simulink model "model"  (R2021b)
settings: Solver=FixedStepAuto  StartTime=0.0  StopTime=100  FixedStep=0.05  RelTol=1e-3
undefined symbols (not defined in the file): A, parameters, waypoints, waypoints_K
libraries: mssSimulink x9
settings Model: Creator=simengangstad  LastModifiedBy=simengangstad

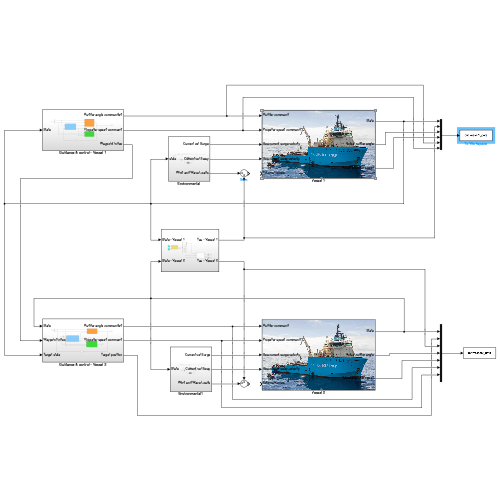
[thumbnail: Simulink's stored preview of the top-level diagram]
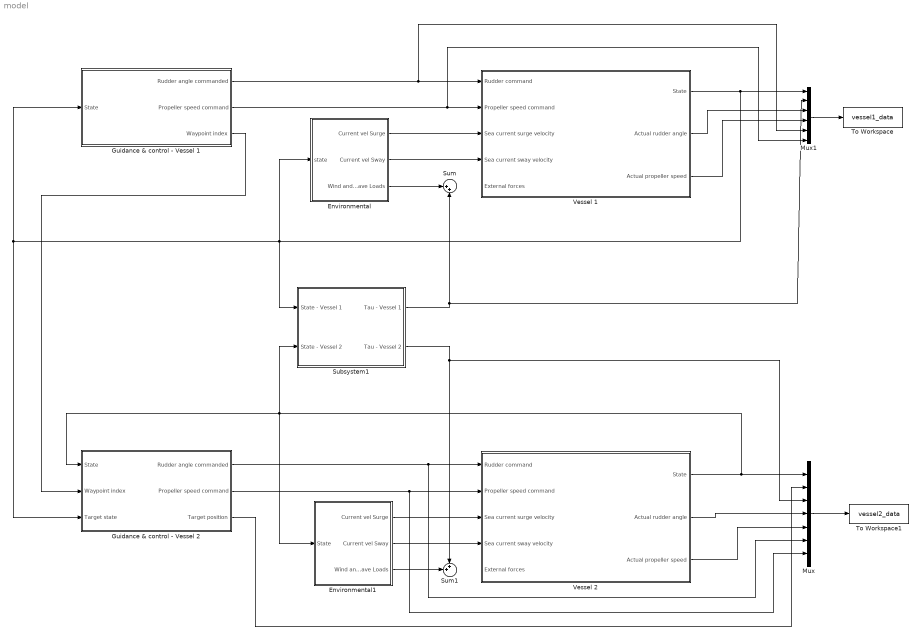
== system model ==
  Environmental : Subsystem
  Environmental1 : Subsystem
  Guidance & control - Vessel 1 : Subsystem
  Guidance & control - Vessel 2 : Subsystem
  Mux : Mux  Inputs=7
  Mux1 : Mux  Inputs=6
  Subsystem1 : Subsystem
  Sum : Sum  Inputs=|++
  Sum1 : Sum  Inputs=++|
  To Workspace : ToWorkspace  VariableName=vessel1_data  SaveFormat=Timeseries  SampleTime=-1
  To Workspace1 : ToWorkspace  VariableName=vessel2_data  SaveFormat=Timeseries  SampleTime=-1
  Vessel 1 : Subsystem
      mask Display: image('$imagefile'); % Use "Edit Image" on toolstrip to change.
  Vessel 2 : Subsystem
      mask Display: image('$imagefile'); % Use "Edit Image" on toolstrip to change.
  wires:
  Vessel 1/1(State) -> Environmental/1(state), Guidance & control - Vessel 1/1(State), Guidance & control - Vessel 2/3(Target state), Subsystem1/1(State - Vessel 1), Mux1/1
  Vessel 1/2(Actual rudder angle) -> Mux1/3
  Vessel 1/3(Actual propeller speed) -> Mux1/4
  Environmental/2(Current vel Sway) -> Vessel 1/4(Sea current sway velocity)
  Environmental/1(Current vel Surge) -> Vessel 1/3(Sea current surge velocity)
  Environmental1/1(Current vel Surge) -> Vessel 2/3(Sea current surge velocity)
  Environmental1/2(Current vel Sway) -> Vessel 2/4(Sea current sway velocity)
  Vessel 2/2(Actual rudder angle) -> Mux/4
  Vessel 2/3(Actual propeller speed) -> Mux/5
  Mux/1 -> To Workspace1/1
  Guidance & control - Vessel 1/1(Rudder angle commanded) -> Mux1/5, Vessel 1/1(Rudder command)
  Guidance & control - Vessel 1/2(Propeller speed command) -> Mux1/6, Vessel 1/2(Propeller speed command)
  Guidance & control - Vessel 1/3(Waypoint index) -> Guidance & control - Vessel 2/2(Waypoint index)
  Guidance & control - Vessel 2/1(Rudder angle commanded) -> Mux/6, Vessel 2/1(Rudder command)
  Guidance & control - Vessel 2/2(Propeller speed command) -> Mux/7, Vessel 2/2(Propeller speed command)
  Guidance & control - Vessel 2/3(Target position) -> Mux/2
  Vessel 2/1(State) -> Subsystem1/2(State - Vessel 2), Guidance & control - Vessel 2/1(State), Environmental1/1(State), Mux/1
  Subsystem1/1(Tau - Vessel 1) -> Sum/2, Mux1/2
  Environmental/3(Wind and Wave Loads) -> Sum/1
  Environmental1/3(Wind and Wave Loads) -> Sum1/2
  Subsystem1/2(Tau - Vessel 2) -> Sum1/1, Mux/3
  Mux1/1 -> To Workspace/1

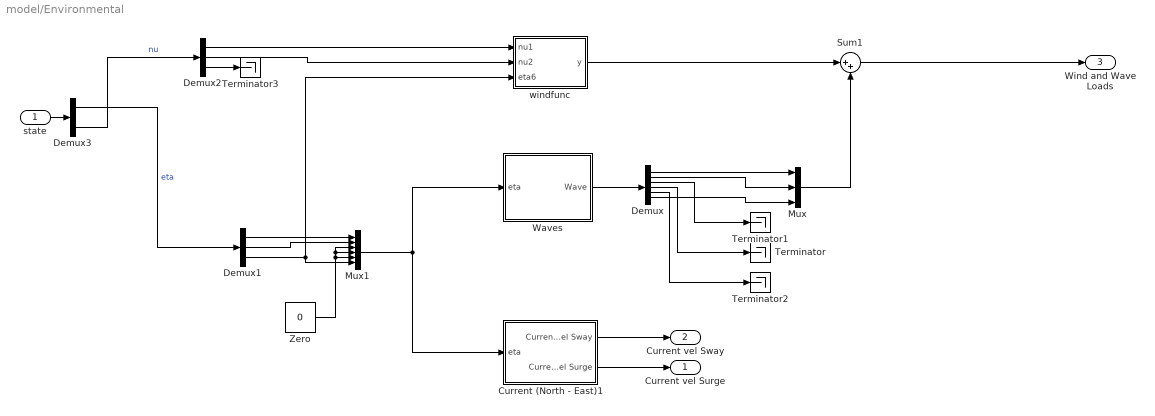
== system model/Environmental ==
  state : Inport
  Current (North - East)1 : Subsystem
  Demux : Demux  Outputs=6
  Demux1 : Demux  Outputs=3
  Demux2 : Demux  Outputs=3
  Demux3 : Demux  Outputs=2
  Mux : Mux  Inputs=3
  Mux1 : Mux  Inputs=6
  Sum1 : Sum  Inputs=|++
  Terminator{,1..3} (4 alike) : Terminator
  Waves : Subsystem
  Zero : Constant  Value=0  OutDataTypeStr=Inherit: Inherit via back propagation
  windfunc : MATLAB Function  TreatAsAtomicUnit=on
  Current vel Surge : Outport
  Current vel Sway : Outport  Port=2
  Wind and Wave Loads : Outport  Port=3
  wires:
  Demux/1 -> Mux/1
  Demux/2 -> Mux/2
  Demux/6 -> Mux/3
  Demux/3 -> Terminator1/1
  Demux/4 -> Terminator/1
  Demux/5 -> Terminator2/1
  Demux3/1 -> Demux1/1  "eta"
  Demux1/1 -> Mux1/1
  Demux1/2 -> Mux1/2
  Demux1/3 -> Mux1/6, windfunc/3(eta6)
  Zero/1 -> Mux1/5, Mux1/4, Mux1/3
  Mux1/1 -> Current (North - East)1/1(eta), Waves/1(eta)
  Waves/1(Wave) -> Demux/1
  windfunc/1(y) -> Sum1/1
  Demux3/2 -> Demux2/1  "nu"
  Demux2/1 -> windfunc/1(nu1)
  Demux2/2 -> windfunc/2(nu2)
  Demux2/3 -> Terminator3/1
  Mux/1 -> Sum1/2
  Sum1/1 -> Wind and Wave Loads/1
  Current (North - East)1/1(Currentvel Sway) -> Current vel Sway/1
  Current (North - East)1/2(Currentvel Surge) -> Current vel Surge/1
  state/1 -> Demux3/1

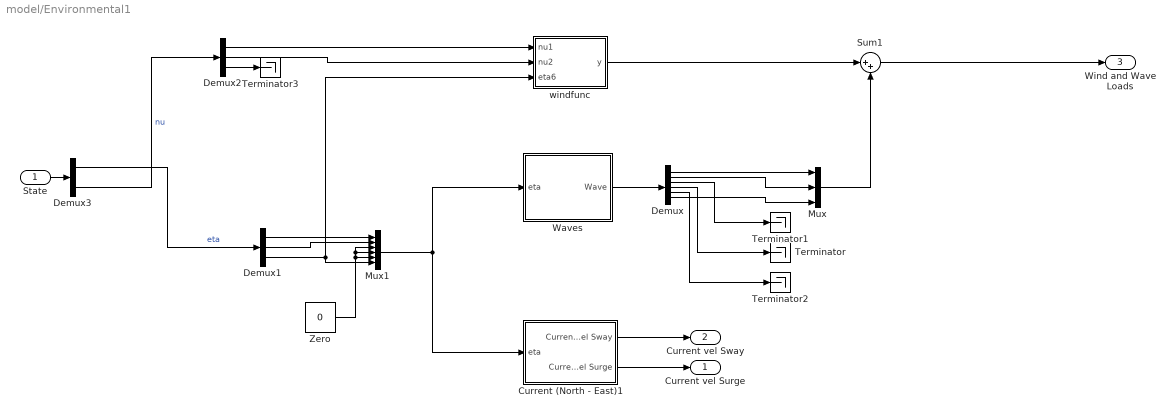
== system model/Environmental1 ==
  State : Inport
  Current (North - East)1 : Subsystem
  Demux : Demux  Outputs=6
  Demux1 : Demux  Outputs=3
  Demux2 : Demux  Outputs=3
  Demux3 : Demux  Outputs=2
  Mux : Mux  Inputs=3
  Mux1 : Mux  Inputs=6
  Sum1 : Sum  Inputs=|++
  Terminator{,1..3} (4 alike) : Terminator
  Waves : Subsystem
  Zero : Constant  Value=0  OutDataTypeStr=Inherit: Inherit via back propagation
  windfunc : MATLAB Function  TreatAsAtomicUnit=on
  Current vel Surge : Outport
  Current vel Sway : Outport  Port=2
  Wind and Wave Loads : Outport  Port=3
  wires:
  Demux/1 -> Mux/1
  Demux/2 -> Mux/2
  Demux/6 -> Mux/3
  Demux/3 -> Terminator1/1
  Demux/4 -> Terminator/1
  Demux/5 -> Terminator2/1
  Demux3/1 -> Demux1/1  "eta"
  Demux1/1 -> Mux1/1
  Demux1/2 -> Mux1/2
  Demux1/3 -> Mux1/6, windfunc/3(eta6)
  Zero/1 -> Mux1/5, Mux1/4, Mux1/3
  Mux1/1 -> Current (North - East)1/1(eta), Waves/1(eta)
  Waves/1(Wave) -> Demux/1
  windfunc/1(y) -> Sum1/1
  Demux3/2 -> Demux2/1  "nu"
  Demux2/1 -> windfunc/1(nu1)
  Demux2/2 -> windfunc/2(nu2)
  Demux2/3 -> Terminator3/1
  Mux/1 -> Sum1/2
  Sum1/1 -> Wind and Wave Loads/1
  Current (North - East)1/1(Currentvel Sway) -> Current vel Sway/1
  Current (North - East)1/2(Currentvel Surge) -> Current vel Surge/1
  State/1 -> Demux3/1

== system model/Guidance & control - Vessel 1 ==
  State : Inport
  Constant : Constant  Value=1.5
  Demux1 : Demux  Outputs=2
  Guidance : Subsystem
  Heading controller : Subsystem
  Memory : Memory
  Speed controller : Subsystem
  Rudder angle commanded : Outport
  Propeller speed command : Outport  Port=2
  Waypoint index : Outport  Port=3
  wires:
  Demux1/2 -> Speed controller/2(nu), Heading controller/2(nu)
  Guidance/2(Waypoint index) -> Waypoint index/1, Speed controller/3(Waypoint index)
  Speed controller/1(Propeller speed command) -> Propeller speed command/1
  Constant/1 -> Speed controller/1(Speed reference)
  Guidance/1(psi_ref) -> Heading controller/3(psi_ref)
  Demux1/1 -> Guidance/1(eta), Heading controller/1(eta)
  Memory/1 -> Guidance/2(Rudder angle commanded)
  Heading controller/1(Rudder angle commanded) -> Rudder angle commanded/1, Memory/1
  State/1 -> Demux1/1

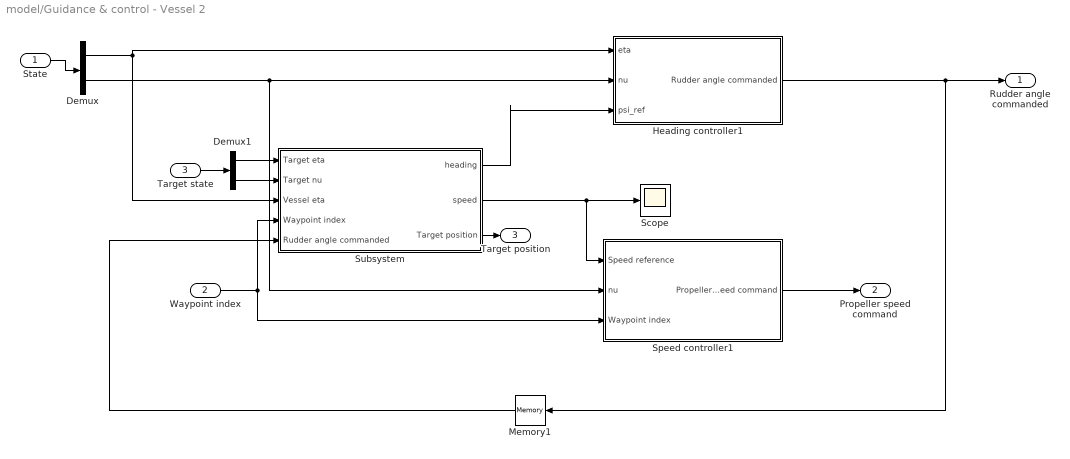
== system model/Guidance & control - Vessel 2 ==
  State : Inport
  Waypoint index : Inport  Port=2
  Target state : Inport  Port=3
  Demux : Demux  Outputs=2
  Demux1 : Demux  Outputs=2
  Heading controller1 : Subsystem
  Memory1 : Memory
  Scope : Scope
  Speed controller1 : Subsystem
  Subsystem : Subsystem
  Rudder angle commanded : Outport
  Propeller speed command : Outport  Port=2
  Target position : Outport  Port=3
  wires:
  Demux1/2 -> Subsystem/2(Target nu)
  Demux1/1 -> Subsystem/1(Target eta)
  Speed controller1/1(Propeller speed command) -> Propeller speed command/1
  Subsystem/3(Target position) -> Target position/1
  Waypoint index/1 -> Subsystem/4(Waypoint index), Speed controller1/3(Waypoint index)
  Memory1/1 -> Subsystem/5(Rudder angle commanded)
  Subsystem/2(speed) -> Scope/1, Speed controller1/1(Speed reference)
  Demux/1 -> Heading controller1/1(eta), Subsystem/3(Vessel eta)
  Subsystem/1(heading) -> Heading controller1/3(psi_ref)
  Demux/2 -> Heading controller1/2(nu), Speed controller1/2(nu)
  Heading controller1/1(Rudder angle commanded) -> Memory1/1, Rudder angle commanded/1
  State/1 -> Demux/1
  Target state/1 -> Demux1/1

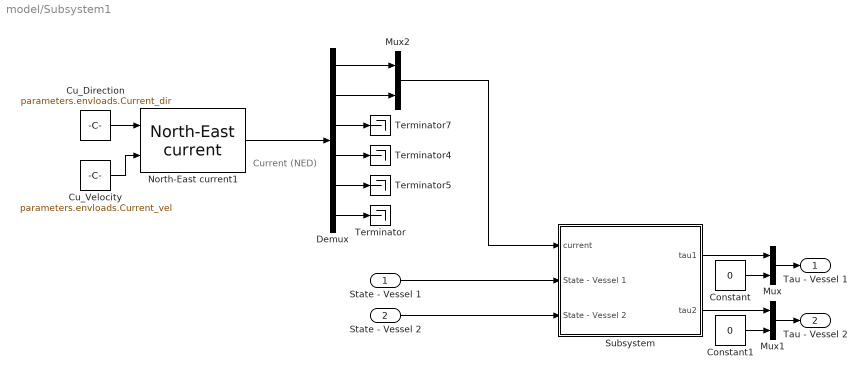
== system model/Subsystem1 ==
  note: Current (NED)
  State - Vessel 1 : Inport
  State - Vessel 2 : Inport  Port=2
  Constant : Constant  Value=0
  Constant1 : Constant  Value=0
  Cu_Direction : Constant  Value=parameters.envloads.Current_dir
  Cu_Velocity : Constant  Value=parameters.envloads.Current_vel
  Demux : Demux  Outputs=6
  Mux : Mux  Inputs=2
  Mux1 : Mux  Inputs=2
  Mux2 : Mux  Inputs=2
  North-East current1 : mssSimulink/Environment/Current/North-East current  SystemSampleTime=-1  VariantActivationTime=update diagram  Latency=0  AutoFrameSizeCalculation=off
  Subsystem : Subsystem
  Terminator{,4..5,7} (4 alike) : Terminator
  Tau - Vessel 1 : Outport
  Tau - Vessel 2 : Outport  Port=2
  wires:
  Demux/6 -> Terminator/1
  Demux/4 -> Terminator4/1
  Demux/1 -> Mux2/1
  North-East current1/1 -> Demux/1
  State - Vessel 1/1 -> Subsystem/2(State - Vessel 1)
  Cu_Direction/1 -> North-East current1/1
  State - Vessel 2/1 -> Subsystem/3(State - Vessel 2)
  Demux/3 -> Terminator7/1
  Mux2/1 -> Subsystem/1(current)
  Cu_Velocity/1 -> North-East current1/2
  Demux/2 -> Mux2/2
  Demux/5 -> Terminator5/1
  Mux/1 -> Tau - Vessel 1/1
  Subsystem/1(tau1) -> Mux/1
  Constant/1 -> Mux/2
  Mux1/1 -> Tau - Vessel 2/1
  Subsystem/2(tau2) -> Mux1/1
  Constant1/1 -> Mux1/2

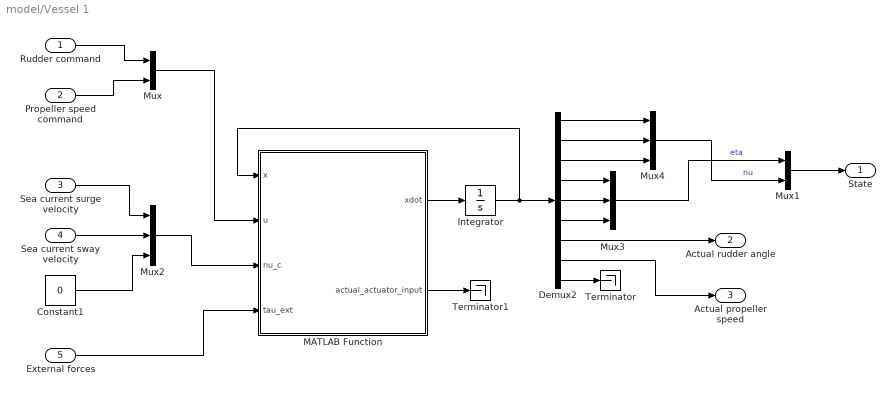
== system model/Vessel 1 ==
  Rudder command : Inport
  Propeller speed command : Inport  Port=2
  Sea current surge velocity : Inport  Port=3
  Sea current sway velocity : Inport  Port=4
  External forces : Inport  Port=5
  Constant1 : Constant  Value=0
  Demux2 : Demux  Outputs=9
  Integrator : Integrator  InitialCondition=[0, 0, 0, 0, 0, pi/2, 0, 0, 0]
  MATLAB Function : MATLAB Function  TreatAsAtomicUnit=on
  Mux : Mux  Inputs=2
  Mux1 : Mux  Inputs=2
  Mux2 : Mux  Inputs=3
  Mux3 : Mux  Inputs=3
  Mux4 : Mux  Inputs=3
  Terminator : Terminator
  Terminator1 : Terminator
  State : Outport
  Actual rudder angle : Outport  Port=2
  Actual propeller speed : Outport  Port=3
  wires:
  Demux2/3 -> Mux4/3
  Demux2/7 -> Actual rudder angle/1
  Mux/1 -> MATLAB Function/2(u)
  External forces/1 -> MATLAB Function/4(tau_ext)
  Mux2/1 -> MATLAB Function/3(nu_c)
  Mux4/1 -> Mux1/2  "nu"
  MATLAB Function/1(xdot) -> Integrator/1
  Propeller speed command/1 -> Mux/2
  Demux2/4 -> Mux3/1
  Demux2/5 -> Mux3/2
  Sea current surge velocity/1 -> Mux2/1
  Constant1/1 -> Mux2/3
  Sea current sway velocity/1 -> Mux2/2
  Mux3/1 -> Mux1/1  "eta"
  Demux2/2 -> Mux4/2
  Demux2/8 -> Actual propeller speed/1
  Demux2/1 -> Mux4/1
  Integrator/1 -> MATLAB Function/1(x), Demux2/1
  Rudder command/1 -> Mux/1
  Demux2/6 -> Mux3/3
  Demux2/9 -> Terminator/1
  MATLAB Function/2(actual_actuator_input) -> Terminator1/1
  Mux1/1 -> State/1

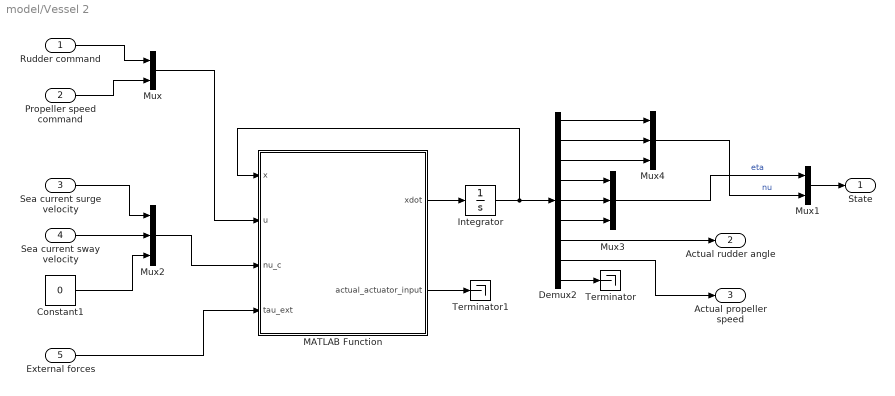
== system model/Vessel 2 ==
  Rudder command : Inport
  Propeller speed command : Inport  Port=2
  Sea current surge velocity : Inport  Port=3
  Sea current sway velocity : Inport  Port=4
  External forces : Inport  Port=5
  Constant1 : Constant  Value=0
  Demux2 : Demux  Outputs=9
  Integrator : Integrator  InitialCondition=[0, 0, 0, 500, 0, pi/2, 0, 0, 0]
  MATLAB Function : MATLAB Function  TreatAsAtomicUnit=on
  Mux : Mux  Inputs=2
  Mux1 : Mux  Inputs=2
  Mux2 : Mux  Inputs=3
  Mux3 : Mux  Inputs=3
  Mux4 : Mux  Inputs=3
  Terminator : Terminator
  Terminator1 : Terminator
  State : Outport
  Actual rudder angle : Outport  Port=2
  Actual propeller speed : Outport  Port=3
  wires:
  Demux2/3 -> Mux4/3
  Demux2/7 -> Actual rudder angle/1
  Mux/1 -> MATLAB Function/2(u)
  External forces/1 -> MATLAB Function/4(tau_ext)
  Mux2/1 -> MATLAB Function/3(nu_c)
  Mux4/1 -> Mux1/2  "nu"
  MATLAB Function/1(xdot) -> Integrator/1
  Propeller speed command/1 -> Mux/2
  Demux2/4 -> Mux3/1
  Demux2/5 -> Mux3/2
  Sea current surge velocity/1 -> Mux2/1
  Constant1/1 -> Mux2/3
  Sea current sway velocity/1 -> Mux2/2
  Mux3/1 -> Mux1/1  "eta"
  Demux2/2 -> Mux4/2
  Demux2/8 -> Actual propeller speed/1
  Demux2/1 -> Mux4/1
  Integrator/1 -> MATLAB Function/1(x), Demux2/1
  Rudder command/1 -> Mux/1
  Demux2/6 -> Mux3/3
  Demux2/9 -> Terminator/1
  MATLAB Function/2(actual_actuator_input) -> Terminator1/1
  Mux1/1 -> State/1

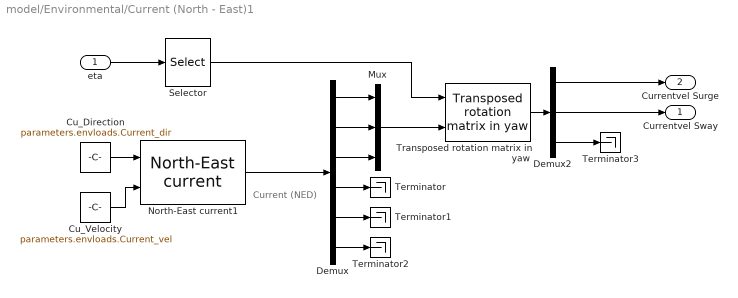
== system model/Environmental/Current (North - East)1 ==
  note: Current (NED)
  eta : Inport
  Cu_Direction : Constant  Value=parameters.envloads.Current_dir
  Cu_Velocity : Constant  Value=parameters.envloads.Current_vel
  Demux : Demux  Outputs=6
  Demux2 : Demux  Outputs=3
  Mux : Mux  Inputs=3
  North-East current1 : mssSimulink/Environment/Current/North-East current  SystemSampleTime=-1  VariantActivationTime=update diagram  Latency=0  AutoFrameSizeCalculation=off
  Selector : Selector  InputPortWidth=6  IndexOptions=Index vector (dialog)  Indices=[6]  OutputSizes=1
  Terminator{,1..3} (4 alike) : Terminator
  Transposed rotation matrix in yaw : mssSimulink/Modelling/Kinematics/Transposed rotation  matrix in yaw
  Currentvel Sway : Outport  VectorParamsAs1DForOutWhenUnconnected=off
  Currentvel Surge : Outport  Port=2
  wires:
  Demux/6 -> Terminator2/1
  North-East current1/1 -> Demux/1
  Demux/4 -> Terminator/1
  Demux/5 -> Terminator1/1
  Selector/1 -> Transposed rotation matrix in yaw/1
  Demux/3 -> Mux/3
  Mux/1 -> Transposed rotation matrix in yaw/2
  Demux/1 -> Mux/1
  Cu_Velocity/1 -> North-East current1/2
  Demux/2 -> Mux/2
  Demux2/2 -> Currentvel Sway/1
  Transposed rotation matrix in yaw/1 -> Demux2/1
  eta/1 -> Selector/1
  Cu_Direction/1 -> North-East current1/1
  Demux2/1 -> Currentvel Surge/1
  Demux2/3 -> Terminator3/1

== system model/Environmental/Waves ==
  eta : Inport
  Terminator : Terminator
  Wave generator : mssSimulink/Environment/Waves/Waves  spectrum_type=ITTC  disp_flag=on  plot_spectrum=off  plot_realization=off  hs=0.8  omega_peak=0  psi_mean=0  gamma=-1  spread=2  depth=inf  nfreq=20  ndir=10  energylim=0.005  freq_cutoff=3  dir_cutoff=0  rand_seed=123  rand_freq=on  rand_dir=on  Zeta_a=0  Omega=0  Phase=0  Wavenum=0  Psi=0
  WaveLoad : Subsystem  mask{waveforces=on}
      mask prompts: waveforces "Waveforces enabled"
  Wave : Outport  VectorParamsAs1DForOutWhenUnconnected=off
  wires:
  Wave generator/1 -> WaveLoad/2(waves)
  Wave generator/2 -> Terminator/1
  eta/1 -> WaveLoad/1(eta)
  WaveLoad/1(Wave) -> Wave/1

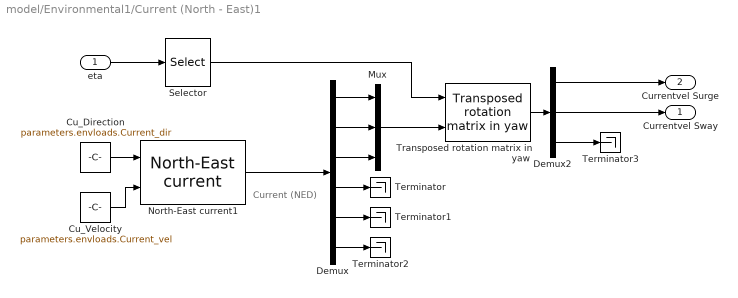
== system model/Environmental1/Current (North - East)1 ==
  note: Current (NED)
  eta : Inport
  Cu_Direction : Constant  Value=parameters.envloads.Current_dir
  Cu_Velocity : Constant  Value=parameters.envloads.Current_vel
  Demux : Demux  Outputs=6
  Demux2 : Demux  Outputs=3
  Mux : Mux  Inputs=3
  North-East current1 : mssSimulink/Environment/Current/North-East current  SystemSampleTime=-1  VariantActivationTime=update diagram  Latency=0  AutoFrameSizeCalculation=off
  Selector : Selector  InputPortWidth=6  IndexOptions=Index vector (dialog)  Indices=[6]  OutputSizes=1
  Terminator{,1..3} (4 alike) : Terminator
  Transposed rotation matrix in yaw : mssSimulink/Modelling/Kinematics/Transposed rotation  matrix in yaw
  Currentvel Sway : Outport  VectorParamsAs1DForOutWhenUnconnected=off
  Currentvel Surge : Outport  Port=2
  wires:
  Demux/6 -> Terminator2/1
  North-East current1/1 -> Demux/1
  Demux/4 -> Terminator/1
  Demux/5 -> Terminator1/1
  Selector/1 -> Transposed rotation matrix in yaw/1
  Demux/3 -> Mux/3
  Mux/1 -> Transposed rotation matrix in yaw/2
  Demux/1 -> Mux/1
  Cu_Velocity/1 -> North-East current1/2
  Demux/2 -> Mux/2
  Demux2/2 -> Currentvel Sway/1
  Transposed rotation matrix in yaw/1 -> Demux2/1
  eta/1 -> Selector/1
  Cu_Direction/1 -> North-East current1/1
  Demux2/1 -> Currentvel Surge/1
  Demux2/3 -> Terminator3/1

== system model/Environmental1/Waves ==
  eta : Inport
  Terminator : Terminator
  Wave generator : mssSimulink/Environment/Waves/Waves  spectrum_type=ITTC  disp_flag=on  plot_spectrum=off  plot_realization=off  hs=0.8  omega_peak=0  psi_mean=0  gamma=-1  spread=2  depth=inf  nfreq=20  ndir=10  energylim=0.005  freq_cutoff=3  dir_cutoff=0  rand_seed=123  rand_freq=on  rand_dir=on  Zeta_a=0  Omega=0  Phase=0  Wavenum=0  Psi=0
  WaveLoad : Subsystem  mask{waveforces=on}
      mask prompts: waveforces "Waveforces enabled"
  Wave : Outport  VectorParamsAs1DForOutWhenUnconnected=off
  wires:
  Wave generator/1 -> WaveLoad/2(waves)
  Wave generator/2 -> Terminator/1
  eta/1 -> WaveLoad/1(eta)
  WaveLoad/1(Wave) -> Wave/1

== system model/Guidance & control - Vessel 1/Guidance ==
  eta : Inport
  Rudder angle commanded : Inport  Port=2
  Demux2 : Demux  Outputs=3
  MATLAB Function : MATLAB Function  TreatAsAtomicUnit=on
  Terminator : Terminator
  psi_ref : Outport
  Waypoint index : Outport  Port=2
  wires:
  MATLAB Function/1(psi_ref) -> psi_ref/1
  eta/1 -> Demux2/1
  Rudder angle commanded/1 -> MATLAB Function/3(rudder_angle_commanded)
  Demux2/1 -> MATLAB Function/1(x)
  Demux2/2 -> MATLAB Function/2(y)
  Demux2/3 -> Terminator/1
  MATLAB Function/2(waypoint_idx) -> Waypoint index/1

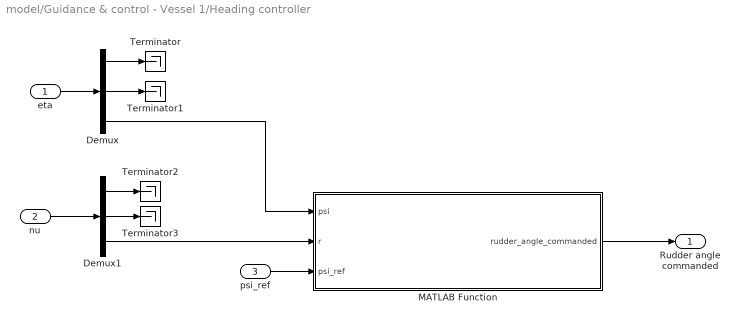
== system model/Guidance & control - Vessel 1/Heading controller ==
  eta : Inport
  nu : Inport  Port=2
  psi_ref : Inport  Port=3
  Demux : Demux  Outputs=3
  Demux1 : Demux  Outputs=3
  MATLAB Function : MATLAB Function  TreatAsAtomicUnit=on
  Terminator{,1..3} (4 alike) : Terminator
  Rudder angle commanded : Outport
  wires:
  MATLAB Function/1(rudder_angle_commanded) -> Rudder angle commanded/1
  Demux1/3 -> MATLAB Function/2(r)
  Demux/2 -> Terminator1/1
  psi_ref/1 -> MATLAB Function/3(psi_ref)
  Demux1/1 -> Terminator2/1
  Demux1/2 -> Terminator3/1
  Demux/3 -> MATLAB Function/1(psi)
  nu/1 -> Demux1/1
  eta/1 -> Demux/1
  Demux/1 -> Terminator/1

== system model/Guidance & control - Vessel 1/Speed controller ==
  Speed reference : Inport
  nu : Inport  Port=2
  Waypoint index : Inport  Port=3
  Demux2 : Demux  Outputs=3
  MATLAB Function : MATLAB Function  TreatAsAtomicUnit=on
  Terminator : Terminator
  Terminator1 : Terminator
  Propeller speed command : Outport
  wires:
  Demux2/1 -> MATLAB Function/1(u)
  Speed reference/1 -> MATLAB Function/2(U_ref)
  nu/1 -> Demux2/1
  MATLAB Function/1(n_c) -> Propeller speed command/1
  Demux2/2 -> Terminator/1
  Demux2/3 -> Terminator1/1
  Waypoint index/1 -> MATLAB Function/3(waypoint_index)

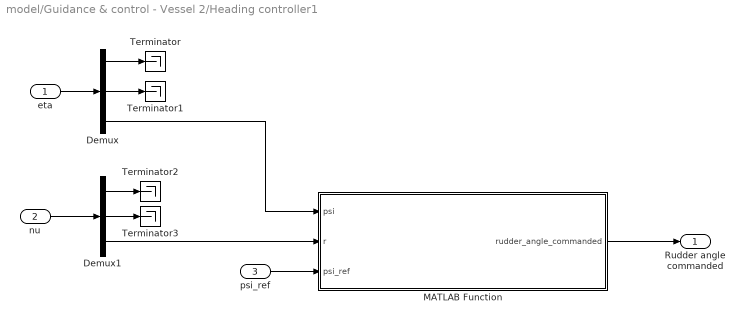
== system model/Guidance & control - Vessel 2/Heading controller1 ==
  eta : Inport
  nu : Inport  Port=2
  psi_ref : Inport  Port=3
  Demux : Demux  Outputs=3
  Demux1 : Demux  Outputs=3
  MATLAB Function : MATLAB Function  TreatAsAtomicUnit=on
  Terminator{,1..3} (4 alike) : Terminator
  Rudder angle commanded : Outport
  wires:
  MATLAB Function/1(rudder_angle_commanded) -> Rudder angle commanded/1
  psi_ref/1 -> MATLAB Function/3(psi_ref)
  Demux1/3 -> MATLAB Function/2(r)
  Demux/3 -> MATLAB Function/1(psi)
  eta/1 -> Demux/1
  nu/1 -> Demux1/1
  Demux/1 -> Terminator/1
  Demux/2 -> Terminator1/1
  Demux1/1 -> Terminator2/1
  Demux1/2 -> Terminator3/1

== system model/Guidance & control - Vessel 2/Speed controller1 ==
  Speed reference : Inport
  nu : Inport  Port=2
  Waypoint index : Inport  Port=3
  Demux2 : Demux  Outputs=3
  MATLAB Function : MATLAB Function  TreatAsAtomicUnit=on
  Terminator : Terminator
  Terminator1 : Terminator
  Propeller speed command : Outport
  wires:
  Demux2/1 -> MATLAB Function/1(u)
  Speed reference/1 -> MATLAB Function/2(U_ref)
  nu/1 -> Demux2/1
  MATLAB Function/1(n_c) -> Propeller speed command/1
  Demux2/2 -> Terminator/1
  Demux2/3 -> Terminator1/1
  Waypoint index/1 -> MATLAB Function/3(waypoint_index)

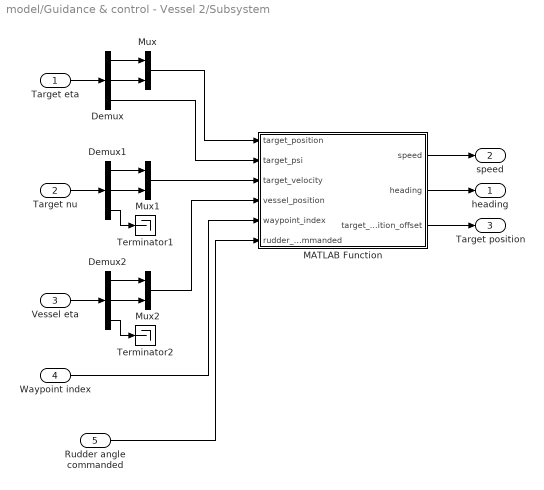
== system model/Guidance & control - Vessel 2/Subsystem ==
  Target eta : Inport
  Target nu : Inport  Port=2
  Vessel eta : Inport  Port=3
  Waypoint index : Inport  Port=4
  Rudder angle commanded : Inport  Port=5
  Demux : Demux  Outputs=3
  Demux1 : Demux  Outputs=3
  Demux2 : Demux  Outputs=3
  MATLAB Function : MATLAB Function  TreatAsAtomicUnit=on
  Mux : Mux  Inputs=2
  Mux1 : Mux  Inputs=2
  Mux2 : Mux  Inputs=2
  Terminator1 : Terminator
  Terminator2 : Terminator
  heading : Outport
  speed : Outport  Port=2
  Target position : Outport  Port=3
  wires:
  MATLAB Function/2(heading) -> heading/1
  MATLAB Function/1(speed) -> speed/1
  Demux/1 -> Mux/1
  Demux/2 -> Mux/2
  Demux/3 -> MATLAB Function/2(target_psi)
  Target eta/1 -> Demux/1
  Mux/1 -> MATLAB Function/1(target_position)
  Mux1/1 -> MATLAB Function/3(target_velocity)
  Demux1/1 -> Mux1/1
  Target nu/1 -> Demux1/1
  Demux1/3 -> Terminator1/1
  Demux1/2 -> Mux1/2
  Vessel eta/1 -> Demux2/1
  Demux2/2 -> Mux2/2
  Demux2/3 -> Terminator2/1
  Demux2/1 -> Mux2/1
  Mux2/1 -> MATLAB Function/4(vessel_position)
  Waypoint index/1 -> MATLAB Function/5(waypoint_index)
  MATLAB Function/3(target_position_offset) -> Target position/1
  Rudder angle commanded/1 -> MATLAB Function/6(rudder_angle_commanded)

== system model/Subsystem1/Subsystem ==
  current : Inport
  State - Vessel 1 : Inport  Port=2
  State - Vessel 2 : Inport  Port=3
  Attack velocity (B frame to net frame) : MATLAB Function  TreatAsAtomicUnit=on
  Demux : Demux  Outputs=2
  Demux1 : Demux  Outputs=2
  Force (net frame to B frame) : MATLAB Function  TreatAsAtomicUnit=on
  Force (net frame) : MATLAB Function  TreatAsAtomicUnit=on
  Net shape : Subsystem
      mask Display: image('$imagefile'); % Use "Edit Image" on toolstrip to change.
  tau1 : Outport
  tau2 : Outport  Port=2
  wires:
  Demux/2 -> Attack velocity (B frame to net frame)/3(nu1)
  Demux1/2 -> Attack velocity (B frame to net frame)/4(nu2)
  Force (net frame)/1(F_x) -> Force (net frame to B frame)/1(F_x)  "F_x"
  Demux1/1 -> Net shape/2(eta2), Attack velocity (B frame to net frame)/2(eta2)
  Force (net frame to B frame)/1(tau1) -> tau1/1  "tau1"
  Demux/1 -> Net shape/1(eta1), Attack velocity (B frame to net frame)/1(eta1)
  Net shape/1(a) -> Force (net frame)/3(a)  "a"
  Attack velocity (B frame to net frame)/1(nu_x) -> Force (net frame)/1(nu_x)  "nu_x"
  Attack velocity (B frame to net frame)/4(r2) -> Force (net frame to B frame)/4(r2)  "r2"
  Net shape/2(distance) -> Force (net frame)/4(span)  "span"
  current/1 -> Attack velocity (B frame to net frame)/5(current)
  Attack velocity (B frame to net frame)/2(nu_y) -> Force (net frame)/2(nu_y)  "nu_y"
  Force (net frame)/2(F_y) -> Force (net frame to B frame)/2(F_y)  "F_y"
  Force (net frame to B frame)/2(tau2) -> tau2/1  "tau2"
  Attack velocity (B frame to net frame)/3(r1) -> Force (net frame to B frame)/3(r1)  "r1"
  State - Vessel 1/1 -> Demux/1
  State - Vessel 2/1 -> Demux1/1

== system model/Environmental/Waves/WaveLoad ==
  eta : Inport
  waves : Inport  Port=2
  Gain : Gain  Gain=waveforces
  Sum : Sum
  Wave loads (U=0) : mssSimulink/Hydrodynamics/Wave loads (U=0)  SystemSampleTime=-1  VariantActivationTime=update diagram  Latency=0  AutoFrameSizeCalculation=off
  Wave : Outport  VectorParamsAs1DForOutWhenUnconnected=off
  wires:
  eta/1 -> Wave loads (U=0)/1
  waves/1 -> Wave loads (U=0)/2
  Sum/1 -> Gain/1
  Wave loads (U=0)/1 -> Sum/1
  Wave loads (U=0)/2 -> Sum/2
  Gain/1 -> Wave/1

== system model/Environmental1/Waves/WaveLoad ==
  eta : Inport
  waves : Inport  Port=2
  Gain : Gain  Gain=waveforces
  Sum : Sum
  Wave loads (U=0) : mssSimulink/Hydrodynamics/Wave loads (U=0)  SystemSampleTime=-1  VariantActivationTime=update diagram  Latency=0  AutoFrameSizeCalculation=off
  Wave : Outport  VectorParamsAs1DForOutWhenUnconnected=off
  wires:
  eta/1 -> Wave loads (U=0)/1
  waves/1 -> Wave loads (U=0)/2
  Sum/1 -> Gain/1
  Wave loads (U=0)/1 -> Sum/1
  Wave loads (U=0)/2 -> Sum/2
  Gain/1 -> Wave/1

== system model/Subsystem1/Subsystem/Net shape ==
  eta1 : Inport
  eta2 : Inport  Port=2
  Prelookup : PreLookup  BreakpointsData=[200:10:750]  ExtrapMethod=Linear
  computing a : Interpolation_n-D  NumberOfTableDimensions=1  Table=A  InternalRulePriority=Speed
      settings: InputPortMap=u0,u1
  span : MATLAB Function  TreatAsAtomicUnit=on
  a : Outport
  distance : Outport  Port=2
  wires:
  eta1/1 -> span/1(eta1)
  Prelookup/1 -> computing a/1
  eta2/1 -> span/2(eta2)
  Prelookup/2 -> computing a/2
  computing a/1 -> a/1
  span/1(span) -> Prelookup/1, distance/1

== matlab function model/Guidance & control - Vessel 2/Heading controller1/MATLAB Function ==
  settings: updateMethod=DISCRETE  sampleTime=0.05
  data: psi input size=1; r input size=1; psi_ref input size=1; rudder_angle_commanded output size=1; parameters parameter
function rudder_angle_commanded = heading_control(psi, r, psi_ref, parameters)
    % Input: 
    % psi: Heading
    % r: Heading rate
    % psi_ref: Heading reference
    % parameters: Ship parameters
    %
    % rudder_angle_commanded: The desired rudder angle

    persistent psi_ref_x e_psi_int;
    
    if isempty(psi_ref_x)
        psi_ref_x = [0; 0; 0];
    end
    
    if isempty(e_psi_int)
        e_psi_int = 0;
    end

    % The derivative coming from the reference model is the state
    % derivative of the reference model
    psi_ref_x_dot = heading_reference_model(psi_ref_x, psi_ref);

    % We can the extract the desired state for heading (psi)
    % and heading rate (r) from the reference model
    psi_desired = psi_ref_x(1);
    r_desired = psi_ref_x(2);

    % Control law
    e_psi = ssa(psi - psi_desired);
    e_r = ssa(r - r_desired);

    % Now we retrieve the rudder angle command from the heading PID
    rudder_angle_commanded = heading_pid(e_psi, ...
                                         e_r, ...
                                         e_psi_int, ...
                                         parameters.nomoto); 

    % Anti-integrator windup
    if abs(rudder_angle_commanded) <= parameters.rudder.max_angle
        e_psi_int = euler2(e_psi, e_psi_int, parameters.simulation.step_size);
    else
        rudder_angle_commanded = parameters.rudder.max_angle ... 
                                 * sign(rudder_angle_commanded);
    end

    
    % Don't care about the integrator windup for the reference model
    psi_ref_x = euler2(psi_ref_x_dot, psi_ref_x, parameters.simulation.step_size);

== matlab function model/Guidance & control - Vessel 2/Speed controller1/MATLAB Function ==
  settings: updateMethod=DISCRETE  sampleTime=0.05
  data: u input; n_c output; U_ref input; waypoint_index input; parameters parameter; waypoints_K parameter
function n_c = speed_control(u, U_ref, waypoint_index, parameters, waypoints_K)

    persistent e_u_int

    if isempty(e_u_int)
        e_u_int = 0;
    end

    u_desired = U_ref;% + 300 * waypoints_K(waypoint_index);
    e_u = u - u_desired;

    % Here n_c is the rps of the motor (n) commanded 
    n_c = speed_pid(u_desired, e_u, e_u_int, parameters);

    e_u_int = euler2(e_u, e_u_int, parameters.simulation.step_size);

== matlab function model/Guidance & control - Vessel 2/Subsystem/MATLAB Function ==
  settings: updateMethod=DISCRETE
  data: target_position input; target_psi input; speed output size=1; target_velocity input; vessel_position input; waypoint_index input; heading output size=1; parameters parameter; waypoints_K parameter; target_position_offset output size=2; waypoints parameter; rudder_angle_commanded input
function [speed, heading, target_position_offset] = CB(target_position, target_psi, target_velocity, vessel_position, waypoint_index, parameters, waypoints_K, waypoints, rudder_angle_commanded)

    [speed, heading, target_position_offset] = constant_bearing(target_position, target_velocity, target_psi, vessel_position, waypoint_index, rudder_angle_commanded, parameters, waypoints_K, waypoints);

end

== matlab function model/Subsystem1/Subsystem/Attack velocity (B frame to net frame) ==
  data: eta1 input; nu_x output size=19; nu_y output size=19; eta2 input; nu1 input; nu2 input; r1 output size=1; r2 output size=1; current input
function [nu_x, nu_y, r1, r2] = Attack_velocity(eta1, eta2, nu1, nu2, current)
n = 20;
nu_x = zeros(n-1,1);
nu_y = zeros(n-1,1);
psi1 = eta1(3);
psi2 = eta2(3);
eta_d = eta2 - eta1;
alpha = atan2(eta_d(2),eta_d(1)) - pi/2; % net orientation

if abs((psi1+psi2)/2-alpha) > pi/2
    alpha = -alpha;
end

r1 = alpha - psi1;
r2 = alpha - psi2;

B = [cos(r1) sin(r1) 0 0; 
        -sin(r1) cos(r1) 0 0;
        0 0 cos(r2) sin(r2);
        0 0 -sin(r2) cos(r2)];
      
R1 = [cos(psi1), sin(psi1);
          -sin(psi1), cos(psi1)];       
R2 = [cos(psi2), sin(psi2);
          -sin(psi2),cos(psi2)];

nu_c1 = R1*current;
nu_c2 = R2*current;

nu = B * [nu1(1)-nu_c1(1);  % nu1_x
                 nu1(2)-nu_c1(2);  % nu1_y
                 nu2(1)-nu_c2(1);  % nu2_x
                 nu2(2)-nu_c2(2)]; % nu2_y
 for i = 1 : n-1
    delta = [nu(3)-nu(1);
                   nu(4)-nu(2)]/(n-1);
    nu_x(i) = nu(3) - (i-0.5) * delta(1);
    nu_y(i) = nu(4) - (i-0.5) * delta(2);
 end
 
end

== matlab function model/Subsystem1/Subsystem/Force (net frame to B frame) ==
  data: F_x input; tau1 output; F_y input; r1 input; r2 input; tau2 output
function [tau1,tau2] = Transformation(F_x, F_y, r1, r2)
B = [cos(r1) sin(r1) 0 0; 
        -sin(r1) cos(r1) 0 0;
        0 0 cos(r2) sin(r2);
        0 0 -sin(r2) cos(r2)];
drag = -[F_x/2;F_y/2;F_x/2;F_y/2];
tau = inv(B) * drag;
tau1 = tau(1:2);
tau2 = tau(3:4);

== matlab function model/Subsystem1/Subsystem/Force (net frame) ==
  data: nu_x input; F_x output; nu_y input; a input; span input; F_y output
function [F_x, F_y]= Force(nu_x, nu_y, a, span)
n = 20;
rho= 1027;
dep = 3; 
d_w = 2.5e-3; 
L = 50e-3; 
Sn = d_w*(2*L+0.5*d_w)/L^2;
D = 0.5;
draft = 0.2*D;
Cd= 1;
F_x = 0;
F_y = 0;

delta_x = span/(n-1);
X = span/2-0.5*delta_x : -delta_x: -span/2+0.5*delta_x;
 for i = 1 : (n-1)
     k = atan(sinh(X(i)/a));
     beta = atan2(nu_y(i), nu_x(i));
     theta = k + beta;
     kappa = theta - beta;
     V = nu_x(i)/cos(beta);
     C_D = 0.04+(-0.04+0.33*Sn+6.54*Sn^2-4.88*Sn^3)*cos(theta);
     C_L = (-0.05*Sn+2.3*Sn^2-1.76*Sn^3)*sin(2*theta);
     F_d1 = 0.5 * C_D * rho * V * abs(V) * dep * delta_x / cos(k); % net drag
     F_l1 = 0.5 * C_L * rho * V * abs(V) * dep * delta_x / cos(k); % net lift
     F_d = 0.5 * Cd * rho * V * cos(theta) * abs(V * cos(theta)) * 0.2 * draft * delta_x / cos(k); % buyo drag
     
     F_x = F_x + F_d1*cos(beta) + F_l1 * sin(beta) + F_d * cos(kappa); 
     F_y = F_y +  F_d1*sin(beta) - F_l1 *cos(beta) - F_d * sin(kappa);
 end

== matlab function model/Subsystem1/Subsystem/Net shape/span ==
  data: eta1 input; span output; eta2 input
function span = dis(eta1, eta2)
pos1 = eta1(1:2);
pos2 = eta2(1:2);
span = norm(pos1-pos2);

== matlab function model/Guidance & control - Vessel 1/Guidance/MATLAB Function ==
  settings: updateMethod=DISCRETE
  data: x input size=1; y input size=1; rudder_angle_commanded input size=1; psi_ref output; parameters parameter; waypoints parameter; waypoints_K parameter; waypoint_idx output
function [psi_ref, waypoint_idx] = guidance_law(x, y, rudder_angle_commanded, parameters, waypoints, waypoints_K)
    % Input:
    % (x, y): Position
    % delta_c: Commanded rudder angle
    % kappa: 
    % parameters: Ship parameters
    %
    % Output:
    % psi_ref: The heading to hold

    persistent y_int waypoint_index
    
    if isempty(y_int)
        y_int = 0;
    end

    if isempty(waypoint_index)
        waypoint_index = 1;
    end


    [current_waypoint, waypoint_index] = closest_waypoint([x, y], waypoints, waypoint_index);
    
    radius = 1000 * (1 - 175 * waypoints_K(waypoint_index));

    [next_waypoint, found] = find_farthest_point_spanned_by_circle(radius, waypoints, waypoint_index);

    if ~found
        next_waypoint = waypoints(:, waypoint_index + 1)';
    end
    
    next_waypoint = waypoints(:, waypoint_index + 1)';

    [e_y, pi_p] = cross_track_error(next_waypoint(1), ...
                                    next_waypoint(2), ...
                                    current_waypoint(1), ...
                                    current_waypoint(2), ...
                                    x, ...
                                    y);

    look_ahead = parameters.guidance.look_ahead * (1 - 150 * waypoints_K(waypoint_index));

    [psi_desired, y_int_dot] = ilos_guidance(e_y, pi_p, y_int, look_ahead, parameters.guidance.kappa);
    psi_ref = psi_desired;

    % Anti-integrator windup
    if abs(rudder_angle_commanded) <= parameters.rudder.max_angle
        y_int = euler2(y_int_dot, y_int, parameters.simulation.step_size);
    end

    waypoint_idx = waypoint_index;

== matlab function model/Vessel 1/MATLAB Function ==
  data: x input size=9; u input size=2; xdot output size=9; nu_c input size=3; tau_ext input size=3; actual_actuator_input output size=2; parameters parameter
function [xdot, actual_actuator_input] = ship(x, u, nu_c, tau_ext, parameters)
    [xdot, actual_actuator_input] = supply_model(x, u, nu_c, tau_ext, parameters);
end

== matlab function model/Guidance & control - Vessel 1/Heading controller/MATLAB Function ==
  settings: updateMethod=DISCRETE  sampleTime=0.05
  data: psi input size=1; r input size=1; psi_ref input size=1; rudder_angle_commanded output size=1; parameters parameter
function rudder_angle_commanded = heading_control(psi, r, psi_ref, parameters)
    % Input: 
    % psi: Heading
    % r: Heading rate
    % psi_ref: Heading reference
    % parameters: Ship parameters
    %
    % rudder_angle_commanded: The desired rudder angle

    persistent psi_ref_x e_psi_int;
    
    if isempty(psi_ref_x)
        psi_ref_x = [0; 0; 0];
    end
    
    if isempty(e_psi_int)
        e_psi_int = 0;
    end

    % The derivative coming from the reference model is the state
    % derivative of the reference model
    psi_ref_x_dot = heading_reference_model(psi_ref_x, psi_ref);

    % We can the extract the desired state for heading (psi)
    % and heading rate (r) from the reference model
    psi_desired = psi_ref_x(1);
    r_desired = psi_ref_x(2);

    % Control law
    e_psi = ssa(psi - psi_desired);
    e_r = ssa(r - r_desired);

    % Now we retrieve the rudder angle command from the heading PID
    rudder_angle_commanded = heading_pid(e_psi, ...
                                         e_r, ...
                                         e_psi_int, ...
                                         parameters.nomoto); 

    % Anti-integrator windup
    if abs(rudder_angle_commanded) <= parameters.rudder.max_angle
        e_psi_int = euler2(e_psi, e_psi_int, parameters.simulation.step_size);
    else
        rudder_angle_commanded = parameters.rudder.max_angle ... 
                                 * sign(rudder_angle_commanded);
    end

    
    % Don't care about the integrator windup for the reference model
    psi_ref_x = euler2(psi_ref_x_dot, psi_ref_x, parameters.simulation.step_size);

== matlab function model/Guidance & control - Vessel 1/Speed controller/MATLAB Function ==
  settings: updateMethod=DISCRETE  sampleTime=0.05
  data: u input; n_c output; U_ref input; waypoint_index input; parameters parameter; waypoints_K parameter
function n_c = speed_control(u, U_ref, waypoint_index, parameters, waypoints_K)

    persistent e_u_int

    if isempty(e_u_int)
        e_u_int = 0;
    end

    u_desired = U_ref + 300 * waypoints_K(waypoint_index);
    e_u = u - u_desired;

    % Here n_c is the rps of the motor (n) commanded 
    n_c = speed_pid(u_desired, e_u, e_u_int, parameters);

    e_u_int = euler2(e_u, e_u_int, parameters.simulation.step_size);

== matlab function model/Vessel 2/MATLAB Function ==
  data: x input size=9; u input size=2; xdot output size=9; nu_c input size=3; tau_ext input size=3; actual_actuator_input output size=2; parameters parameter
function [xdot, actual_actuator_input] = ship(x, u, nu_c, tau_ext, parameters)
    [xdot, actual_actuator_input] = supply_model(x, u, nu_c, tau_ext, parameters);
end

== matlab function model/Environmental/windfunc ==
  data: nu1 input; nu2 input; eta6 input; y output; parameters parameter
function y = fcn(nu1, nu2, eta6,parameters)

% Wind expressed in NED
%parameters.envloads.Vw = 1;
%parameters.envloads.betaVw = deg2rad(135);
rho_a = 1.247;
cy = 0.95;
cn = 0.15;
A_Lw = 10 * parameters.ship.length;

% Wind velocity in world frame
uw = parameters.envloads.Vw * cos(parameters.envloads.betaVw - eta6); 
vw = parameters.envloads.Vw * sin(parameters.envloads.betaVw - eta6); 

% These are relative to the boat's current velocity
u_rw = nu1 - uw;
v_rw = nu2 - vw;
V_rw = sqrt(u_rw^2 + v_rw^2); 
gamma_rw = -atan2(v_rw, u_rw);

% Turn on wind under simulation to see the effect
Ywind = 0.5 * rho_a * V_rw^2 * cy*sin(gamma_rw) * A_Lw;
Nwind = 0.5 * rho_a * V_rw^2 * cn*sin(2*gamma_rw) * A_Lw*parameters.ship.length;


tau_wind = [0 Ywind Nwind]';


y = tau_wind;

== matlab function model/Environmental1/windfunc ==
  data: nu1 input; nu2 input; eta6 input; y output; parameters parameter
function y = fcn(nu1, nu2, eta6,parameters)

% Wind expressed in NED
%parameters.envloads.Vw = 1;
%parameters.envloads.betaVw = deg2rad(135);
rho_a = 1.247;
cy = 0.95;
cn = 0.15;
A_Lw = 10 * parameters.ship.length;

% Wind velocity in world frame
uw = parameters.envloads.Vw * cos(parameters.envloads.betaVw - eta6); 
vw = parameters.envloads.Vw * sin(parameters.envloads.betaVw - eta6); 

% These are relative to the boat's current velocity
u_rw = nu1 - uw;
v_rw = nu2 - vw;
V_rw = sqrt(u_rw^2 + v_rw^2); 
gamma_rw = -atan2(v_rw, u_rw);

% Turn on wind under simulation to see the effect
Ywind = 0.5 * rho_a * V_rw^2 * cy*sin(gamma_rw) * A_Lw;
Nwind = 0.5 * rho_a * V_rw^2 * cn*sin(2*gamma_rw) * A_Lw*parameters.ship.length;


tau_wind = [0 Ywind Nwind]';


y = tau_wind;
